simulink model "Ejercicio_3_DB"  (R2023a)
settings: Solver=VariableStepAuto  StartTime=0.0  StopTime=7  MaxStep=0.001  MinStep=0.0001  RelTol=1e-3
undefined symbols (not defined in the file): g, g0, K, l, M, m
settings Model: Creator=54115  LastModifiedBy=franc
settings SolverCC: AlgebraicLoopSolver=TrustRegion
settings DebuggingCC: UnconnectedInputMsg=warning  UnconnectedOutputMsg=warning  UnconnectedLineMsg=warning
settings ModelReferenceCC: EnableRefExpFcnMdlSchedulingChecks=on

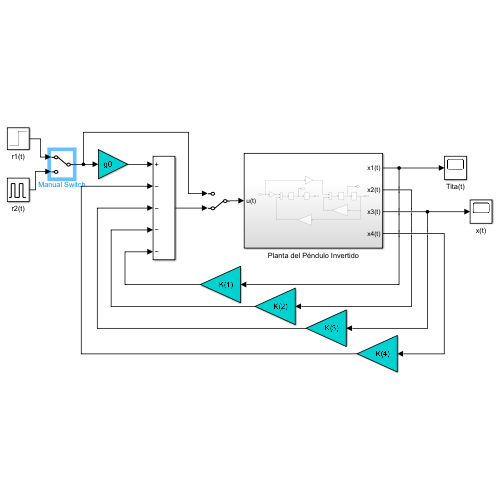
[thumbnail: Simulink's stored preview of the top-level diagram]
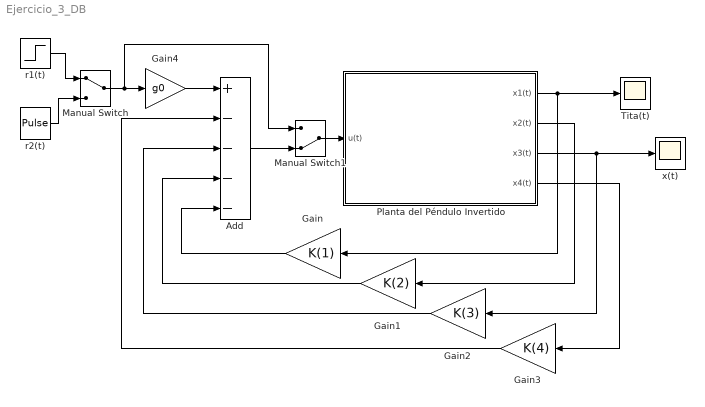
== system Ejercicio_3_DB ==
  Add : Sum  Inputs=+----
  Gain : Gain  Gain=K(1)
  Gain1 : Gain  Gain=K(2)
  Gain2 : Gain  Gain=K(3)
  Gain3 : Gain  Gain=K(4)
  Gain4 : Gain  Gain=g0
  Manual Switch : ManualSwitch
  Manual Switch1 : ManualSwitch  CurrentSetting=0
  Planta del Péndulo Invertido : Subsystem
  "Tita(t) " : Scope
  r1(t) : Step  Time=0  SampleTime=0
  r2(t) : DiscretePulseGenerator  PulseType=Time based  PulseWidth=5
  x(t) : Scope
  wires:
  Planta del Péndulo Invertido/1(x1(t)) -> "Tita(t) "/1, Gain/1
  Planta del Péndulo Invertido/3(x3(t)) -> x(t)/1, Gain2/1
  Planta del Péndulo Invertido/2(x2(t)) -> Gain1/1
  Planta del Péndulo Invertido/4(x4(t)) -> Gain3/1
  Gain/1 -> Add/5
  Gain1/1 -> Add/4
  Gain2/1 -> Add/3
  Gain3/1 -> Add/2
  Gain4/1 -> Add/1
  Manual Switch/1 -> Manual Switch1/1, Gain4/1
  r1(t)/1 -> Manual Switch/1
  r2(t)/1 -> Manual Switch/2
  Manual Switch1/1 -> Planta del Péndulo Invertido/1(u(t))
  Add/1 -> Manual Switch1/2

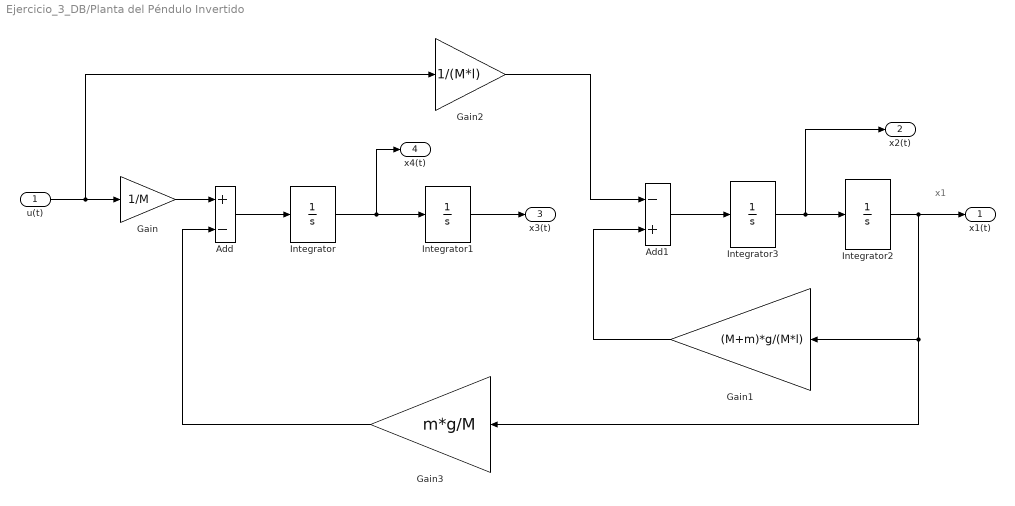
== system Ejercicio_3_DB/Planta del Péndulo Invertido ==
  note: x1
  u(t) : Inport
  Add : Sum  Inputs=+-
  Add1 : Sum  Inputs=-+
  Gain : Gain  Gain=1/M
  Gain1 : Gain  Gain=(M+m)*g/(M*l)
  Gain2 : Gain  Gain=1/(M*l)
  Gain3 : Gain  Gain=m*g/M
  Integrator{,1..3} (4 alike) : Integrator
  x1(t) : Outport
  x2(t) : Outport  Port=2
  x3(t) : Outport  Port=3
  x4(t) : Outport  Port=4
  wires:
  Add/1 -> Integrator/1
  Integrator/1 -> x4(t)/1, Integrator1/1
  Integrator1/1 -> x3(t)/1
  Integrator2/1 -> x1(t)/1, Gain3/1, Gain1/1
  u(t)/1 -> Gain2/1, Gain/1
  Integrator3/1 -> x2(t)/1, Integrator2/1
  Gain1/1 -> Add1/2
  Gain/1 -> Add/1
  Add1/1 -> Integrator3/1
  Gain2/1 -> Add1/1
  Gain3/1 -> Add/2
